simulink model "IIRvariasetapas"  (R2016a)
settings: Solver=VariableStepAuto  StartTime=0.0  StopTime=10.0  RelTol=1e-3
libraries: dspsrcs4 x1
settings Model: SimulationMode=accelerator  Creator=joa-m  LastModifiedBy=joa-m

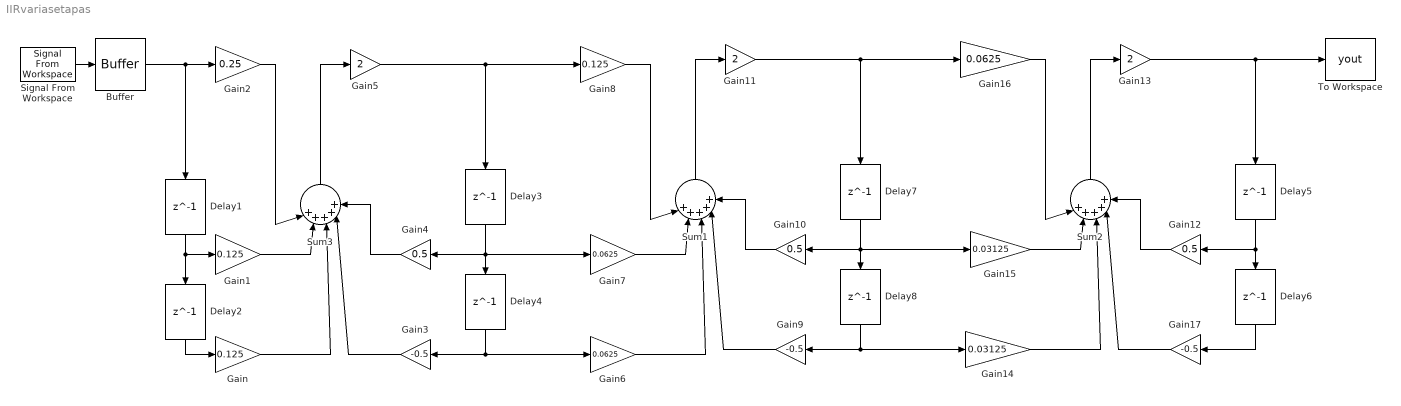
== system IIRvariasetapas ==
  Buffer : Buffer  N=1  TreatMby1Signals=One channel  OutputFrames=off
  Delay{1..8} (8 alike) : Delay  DelayLength=1  InputProcessing=Columns as channels (frame based)
  Gain : Gain  Gain=0.125
  Gain1 : Gain  Gain=0.125
  Gain10 : Gain  Gain=0.5
  Gain11 : Gain  Gain=2
  Gain12 : Gain  Gain=0.5
  Gain13 : Gain  Gain=2
  Gain14 : Gain  Gain=0.03125
  Gain15 : Gain  Gain=0.03125
  Gain16 : Gain  Gain=0.0625
  Gain17 : Gain  Gain=-0.5
  Gain2 : Gain  Gain=0.25
  Gain3 : Gain  Gain=-0.5
  Gain4 : Gain  Gain=0.5
  Gain5 : Gain  Gain=2
  Gain6 : Gain  Gain=0.0625
  Gain7 : Gain  Gain=0.0625
  Gain8 : Gain  Gain=0.125
  Gain9 : Gain  Gain=-0.5
  Signal From Workspace : dspsrcs4/Signal From Workspace  X=[0.5,0,0,0,0]  Ts=1  nsamps=1  OutputAfterFinalValue=Setting to zero  ignoreOrWarnInputAndFrameLengths=off  OutputFrames=off
  Sum1 : Sum  Inputs=|+++++
  Sum2 : Sum  Inputs=|+++++
  Sum3 : Sum  Inputs=|+++++
  To Workspace : ToWorkspace  VariableName=yout  SampleTime=-1
      settings: Save2DSignal=2-D array (concatenate along first dimension)
  wires:
  Signal From Workspace/1 -> Buffer/1
  Delay3/1 -> Gain7/1, Gain4/1, Delay4/1
  Delay4/1 -> Gain6/1, Gain3/1
  Delay2/1 -> Gain/1
  Delay1/1 -> Delay2/1, Gain1/1
  Buffer/1 -> Gain2/1, Delay1/1
  Gain3/1 -> Sum3/4
  Gain/1 -> Sum3/3
  Gain1/1 -> Sum3/2
  Gain2/1 -> Sum3/1
  Gain4/1 -> Sum3/5
  Sum3/1 -> Gain5/1
  Gain5/1 -> Gain8/1, Delay3/1
  Gain9/1 -> Sum1/4
  Gain6/1 -> Sum1/3
  Gain7/1 -> Sum1/2
  Gain8/1 -> Sum1/1
  Gain10/1 -> Sum1/5
  Sum1/1 -> Gain11/1
  Delay7/1 -> Delay8/1, Gain15/1, Gain10/1
  Delay8/1 -> Gain14/1, Gain9/1
  Delay5/1 -> Gain12/1, Delay6/1
  Delay6/1 -> Gain17/1
  Gain11/1 -> Delay7/1, Gain16/1
  Gain17/1 -> Sum2/4
  Gain14/1 -> Sum2/3
  Gain15/1 -> Sum2/2
  Gain16/1 -> Sum2/1
  Gain12/1 -> Sum2/5
  Sum2/1 -> Gain13/1
  Gain13/1 -> To Workspace/1, Delay5/1
